simulink model "rapor_301_2_t10"  (R2020a)
settings: Solver=VariableStepAuto  StartTime=0.0  StopTime=10.0  RelTol=1e-3
settings Model: Creator=nartc  LastModifiedBy=nartc

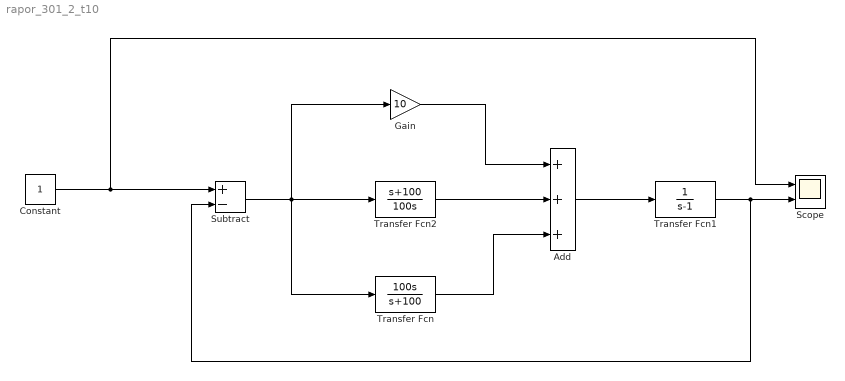
== system rapor_301_2_t10 ==
  Add : Sum  Inputs=+++
  Constant : Constant
  Gain : Gain  Gain=10
  Scope : Scope  NumInputPorts=2
  Subtract : Sum  Inputs=+-
  Transfer Fcn : TransferFcn  Numerator=[100 0]  Denominator=[1 100]
  Transfer Fcn1 : TransferFcn  Denominator=[1 -1]
  Transfer Fcn2 : TransferFcn  Numerator=[1 100]  Denominator=[100 0]
  wires:
  Constant/1 -> Scope/1, Subtract/1
  Gain/1 -> Add/1
  Transfer Fcn/1 -> Add/3
  Transfer Fcn1/1 -> Subtract/2, Scope/2
  Subtract/1 -> Transfer Fcn/1, Gain/1, Transfer Fcn2/1
  Transfer Fcn2/1 -> Add/2
  Add/1 -> Transfer Fcn1/1
